simulink model "hugo_pitch_kalman_sim"  (R2022a)
settings: Solver=VariableStepAuto  StartTime=0.0  StopTime=sim_time  RelTol=1e-3
undefined symbols (not defined in the file or in its folder): est, kalmf
settings Model: Creator=p28ma  LastModifiedBy=hugoa
settings DataIOCC: ReturnWorkspaceOutputs=off
settings DebuggingCC: UnconnectedInputMsg=warning  UnconnectedOutputMsg=warning  UnconnectedLineMsg=warning
settings RTWCC: DLArmComputeVersion=19.05

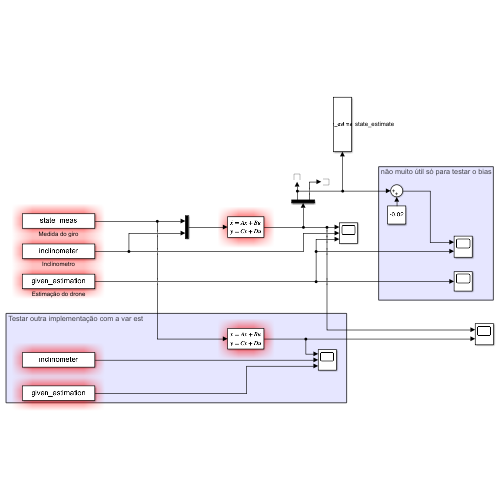
[thumbnail: Simulink's stored preview of the top-level diagram]
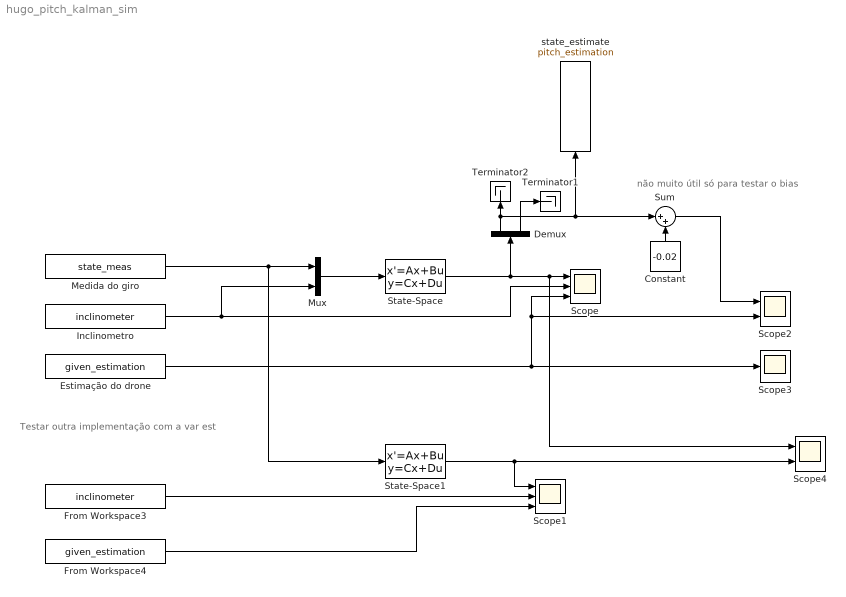
== system hugo_pitch_kalman_sim ==
  note: Testar outra implementação com a var est
  note: não muito útil só para testar o bias
  Constant : Constant  Value=-0.02
  Demux : Demux  Outputs=2
  Estimação do drone : FromWorkspace  VariableName=given_estimation
  From Workspace3 : FromWorkspace  VariableName=inclinometer
  From Workspace4 : FromWorkspace  VariableName=given_estimation
  Inclinometro : FromWorkspace  VariableName=inclinometer
  Medida do giro : FromWorkspace  VariableName=state_meas
  Mux : Mux  Inputs=2
  Scope : Scope  NumInputPorts=3
  Scope1 : Scope  NumInputPorts=3
  Scope2 : Scope  NumInputPorts=2
  Scope3 : Scope
  Scope4 : Scope  NumInputPorts=2
  State-Space : StateSpace  A=kalmf.A  B=kalmf.B  C=kalmf.C  D=kalmf.D  InitialCondition=0
  State-Space1 : StateSpace  A=est.A  B=est.B  C=est.C  D=est.D  InitialCondition=0
  Sum : Sum  Inputs=|++
  Terminator1 : Terminator
  Terminator2 : Terminator
  state_estimate : ToWorkspace  VariableName=pitch_estimation  SaveFormat=Structure With Time  SampleTime=-1
  wires:
  State-Space/1 -> Demux/1, Scope4/1, Scope/1
  State-Space1/1 -> Scope1/1, Scope4/2
  From Workspace4/1 -> Scope1/3
  Mux/1 -> State-Space/1
  Medida do giro/1 -> State-Space1/1, Mux/1
  Demux/2 -> Terminator1/1
  From Workspace3/1 -> Scope1/2
  Demux/1 -> Sum/1, state_estimate/1, Terminator2/1
  Constant/1 -> Sum/2
  Inclinometro/1 -> Mux/2, Scope/2
  Estimação do drone/1 -> Scope2/2, Scope/3, Scope3/1
  Sum/1 -> Scope2/1
